simulink model "dmpRLtest"  (R2018b)
settings: Solver=VariableStepAuto  StartTime=0.0  StopTime=20  RelTol=1e-3
values from neighbouring files (symbols this model uses):
  ankleRollL = mean([modified5times(33,:);modified5times(37,:);modified5times(41,:);modified5times(45,:);modified5times(49,:)])    [dmpRL.m]
  ankleRollR = mean([modified5times(34,:);modified5times(38,:);modified5times(42,:);modified5times(46,:);modified5times(50,:)])    [dmpRL.m]
  arm_radius = leg_radius    (= 0.01)    [Nao_paramter.m]
  foot_height = 0.02    [Nao_paramter.m]
  foot_length = 0.1    [Nao_paramter.m]
  foot_mass = 0.17184    [Nao_paramter.m]
  foot_width = 0.05    [Nao_paramter.m]
  ground_height = 0.0025    [Nao_paramter.m]
  ground_length = 5    [Nao_paramter.m]
  ground_width = 2    [Nao_paramter.m]
  hand_mass = 0.18533    [Nao_paramter.m]
  head_mass = 0.60533    [Nao_paramter.m]
  hip_mass = 0.14053    [Nao_paramter.m]
  hip_off_Y = 0.05    [Nao_paramter.m]
  hip_off_Z = 0.085    [Nao_paramter.m]
  hipRollL = mean([modified5times(31,:);modified5times(35,:);modified5times(39,:);modified5times(43,:);modified5times(47,:)])    [dmpRL.m]
  hipRollR = mean([modified5times(32,:);modified5times(36,:);modified5times(40,:);modified5times(44,:);modified5times(48,:)])    [dmpRL.m]
  leg_radius = 0.01    [Nao_paramter.m]
  lowerarm_length = 0.05595    [Nao_paramter.m]
  lowerarm_mass = 0.07761    [Nao_paramter.m]
  neck_length = 0.03    [Nao_paramter.m]
  neck_mass = 0.07842    [Nao_paramter.m]
  neck_off_Z = 0.1265    [Nao_paramter.m]
  shoulder_mass = 0.09304    [Nao_paramter.m]
  thigh_mass = 0.38968    [Nao_paramter.m]
  tibia_mass = 0.30142    [Nao_paramter.m]
  torso_height = foot_height + tibia_length + thigh_length + 0.5*hip_off_Z    (= 0.2654)    [Nao_paramter.m]
  torso_mass = 1.0496    [Nao_paramter.m]
  upperarm_length = 0.105    [Nao_paramter.m]
  upperarm_mass = 0.15777    [Nao_paramter.m]
undefined symbols (not defined in the file or in its folder): X, Y, Z
libraries: sm_lib x82, nesl_utility x16, simulink x10, Contact_Forces_Lib x10
(part 1 of 4)
settings Model: Creator=Robotarm  LastModifiedBy=zicho

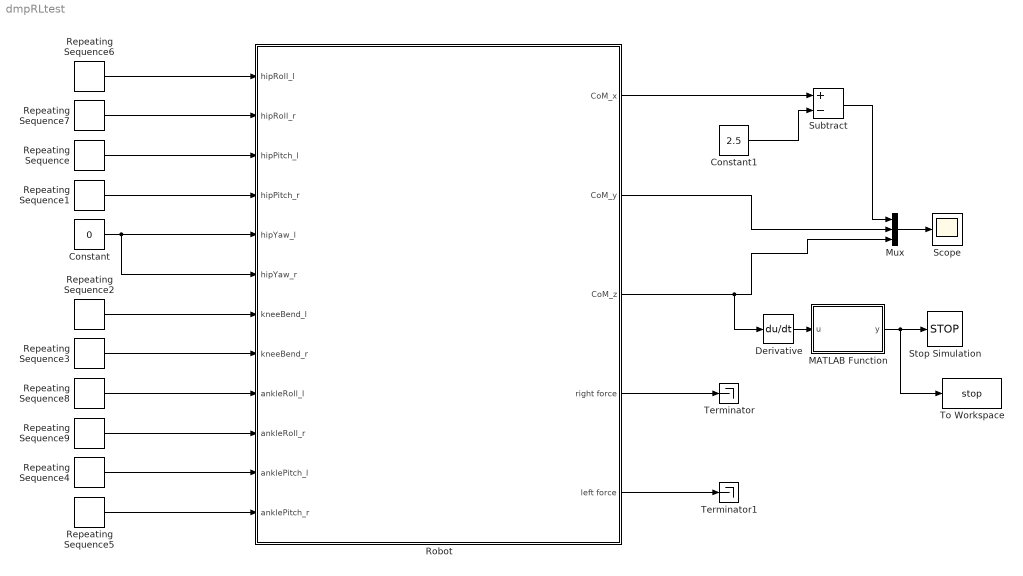
== system dmpRLtest ==
  Constant : Constant  Value=0
  Constant1 : Constant  Value=2.5
  Derivative : Derivative
  MATLAB Function : MATLAB Function  TreatAsAtomicUnit=on
  Mux : Mux  Inputs=3
  Repeating Sequence : simulink/Sources/Repeating Sequence  rep_seq_t=t  rep_seq_y=hipPitchL
  Repeating Sequence1 : simulink/Sources/Repeating Sequence  rep_seq_t=t  rep_seq_y=hipPitchR
  Repeating Sequence2 : simulink/Sources/Repeating Sequence  rep_seq_t=t  rep_seq_y=kneeBendL
  Repeating Sequence3 : simulink/Sources/Repeating Sequence  rep_seq_t=t  rep_seq_y=kneeBendR
  Repeating Sequence4 : simulink/Sources/Repeating Sequence  rep_seq_t=t  rep_seq_y=anklePitchL
  Repeating Sequence5 : simulink/Sources/Repeating Sequence  rep_seq_t=t  rep_seq_y=anklePitchR
  Repeating Sequence6 : simulink/Sources/Repeating Sequence  rep_seq_t=t  rep_seq_y=-hipRollL
  Repeating Sequence7 : simulink/Sources/Repeating Sequence  rep_seq_t=t  rep_seq_y=-hipRollR
  Repeating Sequence8 : simulink/Sources/Repeating Sequence  rep_seq_t=t  rep_seq_y=-ankleRollL
  Repeating Sequence9 : simulink/Sources/Repeating Sequence  rep_seq_t=t  rep_seq_y=-ankleRollR
  Robot : Subsystem
      mask Display: image('multibody.jpg');
  Scope : Scope
  Stop Simulation : Stop
  Subtract : Sum  Inputs=+-
  Terminator : Terminator
  Terminator1 : Terminator
  To Workspace : ToWorkspace  VariableName=stop  SampleTime=0.01
      settings: Save2DSignal=2-D array (concatenate along first dimension)
  wires:
  Robot/4(right force) -> Terminator/1
  Robot/5(left force) -> Terminator1/1
  Constant/1 -> Robot/6(hipYaw_r), Robot/5(hipYaw_l)
  Repeating Sequence4/1 -> Robot/11(anklePitch_l)
  Repeating Sequence5/1 -> Robot/12(anklePitch_r)
  Repeating Sequence8/1 -> Robot/9(ankleRoll_l)
  Repeating Sequence2/1 -> Robot/7(kneeBend_l)
  Mux/1 -> Scope/1
  Repeating Sequence6/1 -> Robot/1(hipRoll_l)
  Repeating Sequence7/1 -> Robot/2(hipRoll_r)
  Repeating Sequence1/1 -> Robot/4(hipPitch_r)
  Robot/2(CoM_y) -> Mux/2
  Repeating Sequence9/1 -> Robot/10(ankleRoll_r)
  Robot/1(CoM_x) -> Subtract/1
  Repeating Sequence3/1 -> Robot/8(kneeBend_r)
  Constant1/1 -> Subtract/2
  Subtract/1 -> Mux/1
  Repeating Sequence/1 -> Robot/3(hipPitch_l)
  Robot/3(CoM_z) -> Derivative/1, Mux/3
  Derivative/1 -> MATLAB Function/1(u)
  MATLAB Function/1(y) -> To Workspace/1, Stop Simulation/1
